simulink model "mtq_deallocation_lib"  (R2018b)
settings: Solver=VariableStepAuto  StartTime=0.0  StopTime=10.0  RelTol=1e-3
settings Model: Creator=Nick's PC  LastModifiedBy=Nick's PC

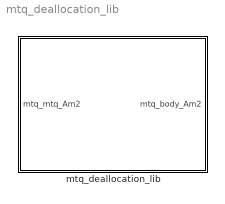
== system mtq_deallocation_lib ==
  mtq_deallocation_lib : Subsystem

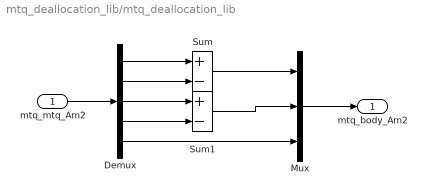
== system mtq_deallocation_lib/mtq_deallocation_lib ==
  mtq_mtq_Am2 : Inport
  Demux : Demux  Outputs=5
  Mux : Mux  Inputs=3
  Sum : Sum  Inputs=+-
  Sum1 : Sum  Inputs=+-
  mtq_body_Am2 : Outport
  wires:
  mtq_mtq_Am2/1 -> Demux/1
  Mux/1 -> mtq_body_Am2/1
  Demux/1 -> Sum/1
  Demux/2 -> Sum/2
  Demux/3 -> Sum1/1
  Demux/4 -> Sum1/2
  Sum/1 -> Mux/1
  Sum1/1 -> Mux/2
  Demux/5 -> Mux/3
